simulink model "validar_espacio_estado_engrane_simulink"  (R2017b)
settings: Solver=VariableStepAuto  StartTime=0.0  StopTime=100  RelTol=1e-3
settings Model: Creator=xmax1  LastModifiedBy=xmax1

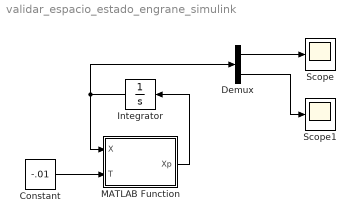
== system validar_espacio_estado_engrane_simulink ==
  Constant : Constant  Value=-.01
  Demux : Demux  Outputs=2
  Integrator : Integrator  InitialCondition=[0 ; 100]
  MATLAB Function : MATLAB Function  TreatAsAtomicUnit=on
  Scope : Scope
  Scope1 : Scope
  wires:
  MATLAB Function/1(Xp) -> Integrator/1
  Integrator/1 -> Demux/1, MATLAB Function/1(X)
  Demux/1 -> Scope/1
  Demux/2 -> Scope1/1
  Constant/1 -> MATLAB Function/2(T)

== matlab function validar_espacio_estado_engrane_simulink/MATLAB Function ==
  data: X input; Xp output; T input
function Xp = engrane(X, T)

J = 1 * 10^-3;
D = 1 * 10^-2;

A = [0, 1 ; 0 -J/D ];
B = [0 ; 1/J];

Xp = A*X + B*T;
